simulink model "exp3_q2"  (R2019a)
settings: Solver=FixedStepAuto  StartTime=0.0  StopTime=3e-1  FixedStep=1e-7  RelTol=1e-3
libraries: dsparch4 x2
settings Model: Creator=marco  LastModifiedBy=marco
settings DebuggingCC: SigSpecEnsureSampleTimeMsg=none

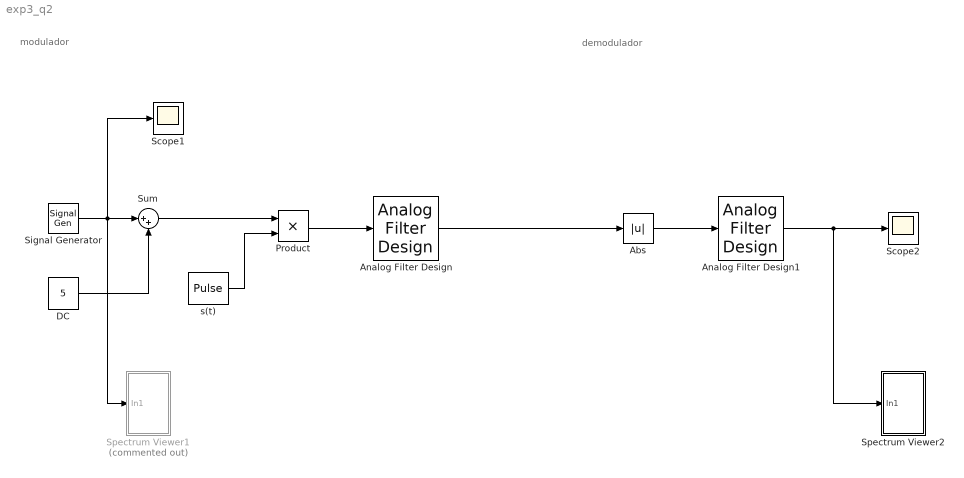
== system exp3_q2 ==
  note: demodulador
  note: modulador
  Abs : Abs
  Analog Filter Design : dsparch4/Analog Filter Design  method=Butterworth  filttype=Bandpass  N=10  Wlo=2*pi*980e3  Whi=2*pi*1020e3  Rp=2  Rs=40
  Analog Filter Design1 : dsparch4/Analog Filter Design  method=Butterworth  filttype=Lowpass  N=10  Wlo=2*pi*2e6  Whi=2*pi*1020e3  Rp=2  Rs=40
  DC : Constant  Value=5
  Product : Product
  Scope1 : Scope
  Scope2 : Scope
  Signal Generator : SignalGenerator  WaveForm=square  Frequency=500
  Spectrum Viewer1 : Subsystem  Commented=on
  Spectrum Viewer2 : Subsystem
  Sum : Sum  Inputs=|++
  "s(t) " : DiscretePulseGenerator  PulseType=Time based  Period=1e-6  PulseWidth=50
  wires:
  Product/1 -> Analog Filter Design/1
  Sum/1 -> Product/1
  Signal Generator/1 -> Scope1/1, Spectrum Viewer1/1(In1), Sum/1
  DC/1 -> Sum/2
  "s(t) "/1 -> Product/2
  Analog Filter Design/1 -> Abs/1
  Abs/1 -> Analog Filter Design1/1
  Analog Filter Design1/1 -> Spectrum Viewer2/1(In1), Scope2/1

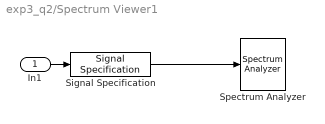
== system exp3_q2/Spectrum Viewer1 ==
  In1 : Inport
  Signal Specification : SignalSpecification  SampleTime=1e-4
  Spectrum Analyzer : SpectrumAnalyzer
  wires:
  In1/1 -> Signal Specification/1
  Signal Specification/1 -> Spectrum Analyzer/1

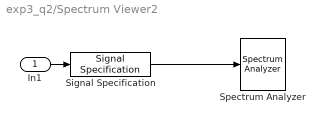
== system exp3_q2/Spectrum Viewer2 ==
  In1 : Inport
  Signal Specification : SignalSpecification  SampleTime=1e-4
  Spectrum Analyzer : SpectrumAnalyzer
  wires:
  In1/1 -> Signal Specification/1
  Signal Specification/1 -> Spectrum Analyzer/1
